simulink model "Lab2Simulink"  (R2014a)
settings: Solver=ode45  StartTime=0.0  StopTime=10.0  RelTol=1e-3
settings Model: Creator=User  LastModifiedBy=User

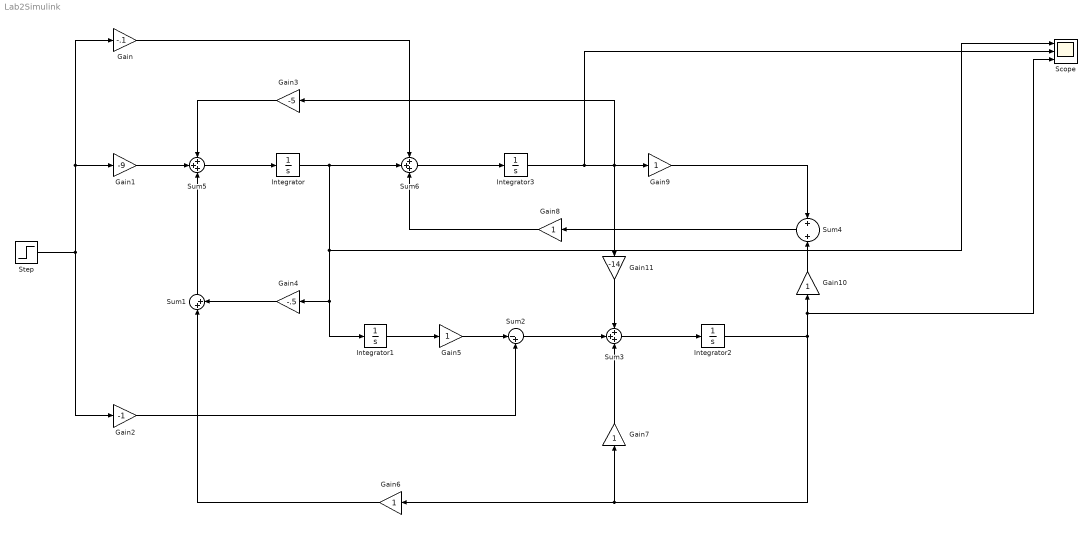
== system Lab2Simulink ==
  Gain : Gain  Gain=-.1
  Gain1 : Gain  Gain=-9
  Gain{5..10} (6 alike) : Gain
  Gain11 : Gain  Gain=-14
  Gain2 : Gain  Gain=-1
  Gain3 : Gain  Gain=-5
  Gain4 : Gain  Gain=-.5
  Integrator{,1..3} (4 alike) : Integrator
  Scope : Scope  NumInputPorts=3
      settings: YMin=-5~-5~-5  YMax=5~5~5
  Step : Step  SampleTime=0
  Sum1 : Sum  Inputs=|++
  Sum2 : Sum  Inputs=|-+
  Sum3 : Sum  Inputs=+++
  Sum4 : Sum
  Sum5 : Sum  Inputs=+++
  Sum6 : Sum  Inputs=+++
  wires:
  Gain3/1 -> Sum5/1
  Gain1/1 -> Sum5/2
  Sum5/1 -> Integrator/1
  Sum1/1 -> Sum5/3
  Gain4/1 -> Sum1/2
  Gain2/1 -> Sum2/2
  Gain6/1 -> Sum1/1
  Gain/1 -> Sum6/1
  Integrator/1 -> Scope/1, Gain4/1, Integrator1/1, Sum6/2
  Gain8/1 -> Sum6/3
  Integrator1/1 -> Gain5/1
  Gain5/1 -> Sum2/1
  Sum6/1 -> Integrator3/1
  Integrator3/1 -> Scope/2, Gain3/1, Gain11/1, Gain9/1
  Gain9/1 -> Sum4/1
  Sum4/1 -> Gain8/1
  Sum2/1 -> Sum3/2
  Gain11/1 -> Sum3/1
  Gain7/1 -> Sum3/3
  Sum3/1 -> Integrator2/1
  Gain10/1 -> Sum4/2
  Integrator2/1 -> Gain7/1, Gain6/1, Scope/3, Gain10/1
  Step/1 -> Gain2/1, Gain1/1, Gain/1
